simulink model "Furuta_Control_2015a"  (R2015a)
settings: Solver=ode3  SolverMode=SingleTasking  StartTime=0.0  StopTime=10  FixedStep=0.0001  RelTol=1e-3
PostLoadFcn:
  | , if any(exist('dsrtsu_mdlpostloadfcn', 'file') == [2, 3, 6]), try dsrtsu_mdlpostloadfcn('Execute', bdroot); catch fprintf('Error in PostLoadFcn (dsrtsu_mdlpostloadfcn) for model "%s":\n %s\n', bdroot, lasterr); end, end,
values from neighbouring files (symbols this model uses):
  alpha = J + (M+m1/3+m2)*L1^2    (= 0.002160093571)    [Furuta_Constants.m]
  beta = (M + m2/3)*L2^2    (= 0.00192796261667)    [Furuta_Constants.m]
  gamma = (M + m2/2)*L2*L1    (= 0.0009263333625)    [Furuta_Constants.m]
  initial_state = pi    (= 3.14159265359)    [Furuta_Constants.m]
  K = place(Ap,Bp,[-7 -5 -3+3j -3-3j])    [Furuta_Constants.m]
  kb = 6e-4    (= 0.0006)    [Furuta_Constants.m]
  ke = 0.182    [Furuta_Constants.m]
  kSU = 0.44    [Furuta_Constants.m]
  Re = 3.6    [Furuta_Constants.m]
  sigma = (M + m2/2)*g*L2    (= 0.0951054975)    [Furuta_Constants.m]
libraries: simulink_extras x1
settings Model: DSRTSU_INTERNAL_RTI_VER=450  DSRTSU_INTERNAL_RTI_TYPE=rti1006  DSRTSU_INTERNAL_RTIFPGA=40  CovMetricSettings=dwe  CovHtmlReporting=off  covSaveCumulativeToWorkspaceVar=off  CovSaveSingleToWorkspaceVar=off  CovExternalEMLEnable=on  Creator=Marcelo  LastModifiedBy=NSEE
settings SolverCC: ZeroCrossControl=DisableAll
settings DataIOCC: LimitDataPoints=off  SaveFormat=Dataset
settings OptimizationCC: BlockReduction=off  OptimizeBlockIOStorage=off  BufferReuse=off  GlobalBufferReuse=off  ExpressionFolding=off  LocalBlockOutputs=off
settings DebuggingCC: ParameterOverflowMsg=warning  SFUnexpectedBacktrackingDiag=error  SFNoUnconditionalDefaultTransitionDiag=error
settings HardwareCC: ProdBitPerPointer=64  ProdLargestAtomicFloat=Float  ProdIntDivRoundTo=Zero  ProdEndianess=LittleEndian  ProdHWDeviceType=Generic->Custom  TargetIntDivRoundTo=Zero  TargetEndianess=LittleEndian  TargetHWDeviceType=Generic->Custom
settings ModelReferenceCC: ModelReferenceMinAlgLoopOccurrences=on  PropagateSignalLabelsOutOfModel=on
settings RTWCC: SystemTargetFile=rti1006.tlc  MakeCommand=make_rti  TemplateMakefile=rti1006.tmf  Description=dSPACE DS1006 Hardware Platform
settings STFCustomTargetCC: GenerateSampleERTMain=off  ParMdlRefBuildCompliant=on  GeneratePreprocessorConditionals=Disable all  ERTCustomFileBanners=off  SupportNonInlinedSFcns=on  SupportVariableSizeSignals=off  MATLABClassNameForMDSCustomization=Simulink.SoftwareTarget.GRTCustomization  GRTInterface=on  SystemTargetFile=rti1006.tlc
settings GRTTargetCC: CompOptLevelCompliant=off  ConcurrentExecutionCompliant=off  CombineOutputUpdateFcns=off  MatFileLogging=off  CPPClassGenCompliant=off  GRTInterface=on  ExtModeMexFile=noextcomm

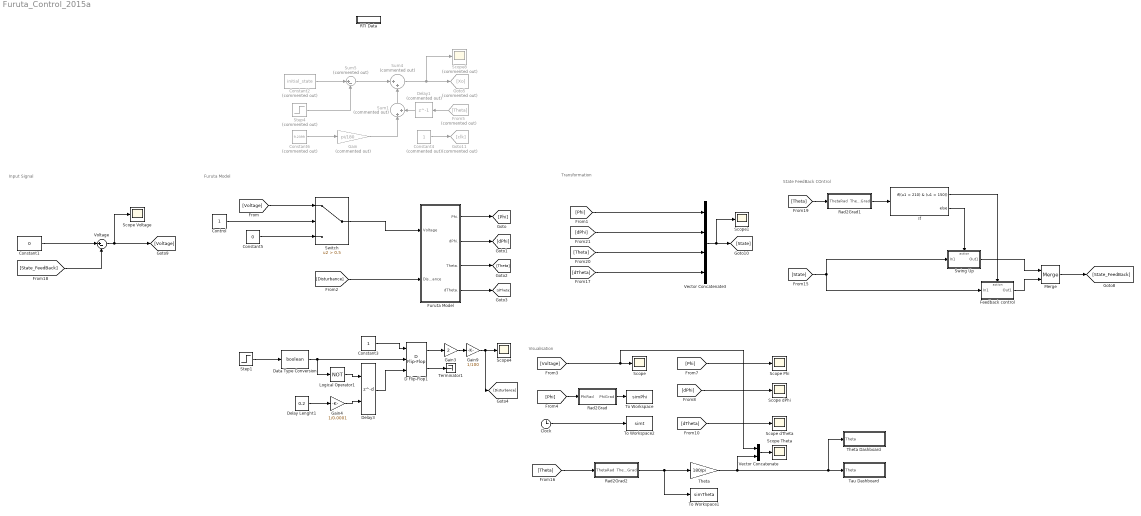
== system Furuta_Control_2015a ==
  note: Transformation
  note: State FeedBack COntrol
  note: Input Signal
  note: Furuta Model
  note: Visualisation
  Clock : Clock
  Constant1 : Constant  Value=0
  Constant2 : Constant  Commented=on  Value=initial_state
  Constant3 : Constant  OutDataTypeStr=boolean
  Constant4 : Constant  Commented=on
  Constant5 : Constant  Value=0
  Constant6 : Constant  Commented=on  Value=9.2399
  Control : Constant
  D Flip-Flop1 : simulink_extras/Flip Flops/D Flip-Flop
  Data Type Conversion : DataTypeConversion  OutDataTypeStr=boolean
  Delay Lenght1 : Constant  Value=0.2  OutDataTypeStr=double
  Delay1 : Delay  Commented=on  DelayLength=1
  Delay3 : Delay  DelayLengthSource=Input port  DelayLengthUpperLimit=100000  InitialCondition=1
      settings: InputPortMap=u0,p1
  Feedback control : Subsystem  TreatAsAtomicUnit=on
  From5 : From  Commented=on  GotoTag=Theta
  "Furuta Model " : Subsystem
  Gain : Gain  Commented=on  Gain=pi/180
  Gain3 : Gain  Gain=2  ParamDataTypeStr=double
  Gain4 : Gain  Gain=1/0.0001
  Gain9 : Gain  Gain=1/100
  Goto11 : Goto  Commented=on  GotoTag=clk
  Goto5 : Goto  Commented=on  GotoTag=Xo
  If : If  IfExpression=(u1 < 210) & (u1 > 150)
  Logical Operator1 : Logic  Operator=NOT  AllPortsSameDT=off  OutDataTypeStr=boolean
  Merge : Merge
  RTI Data : Subsystem  Tag=struct('RTIDataServer',struct('RTIDataServerVs','2','RTIModelDescription','struct(''main'',''Furuta_Control_2015a'',''sub'','''',''isMp'',0)'))  LoadFcn="if exist('rtidc'), try,  rtidc('DataHostBlockClbLoad', gcbh); catch, disp(['Warning: ''LoadFcn'' for RTI Data block failed: ' lasterr]); end, end,"  mask(RTI_DATA_HOST){}
      mask help:
      | RTI Data Block.
      | This block is used by RTI to store internal model-dependent data.
      | Please keep this block on the root level of the model. Deleting this block will result in data loss.
      |
      | NEVER DELETE OR COPY THIS BLOCK!
      settings: CopyFcn="if exist('rtidc'), try,  rtidc('DataHostBlockClbCopy', gcbh); catch, disp(['Warning: ''CopyFcn'' for RTI Data block failed: ' lasterr]); end, end,"  DeleteFcn="if exist('rtidc'), try,  rtidc('DataHostBlockClbDelete', gcbh); catch, disp(['Warning: ''DeleteFcn'' for RTI Data block failed: ' lasterr]); end, end,"  ModelCloseFcn="if exist('rtidc'), try,  rtidc('DataHostBlockClbModelClose', gcbh); catch, disp(['Warning: ''ModelCloseFcn'' for RTI Data block failed: ' lasterr]); end, end,"  PreSaveFcn="if exist('rtidc'), try,  rtidc('DataHostBlockClbPreSave', gcbh); catch, disp(['Warning: ''PreSaveFcn'' for RTI Data block failed: ' lasterr]); end, end,"  PostSaveFcn="if exist('rtidc'), try,  rtidc('DataHostBlockClbPostSave', gcbh); catch, disp(['Warning: ''PostSaveFcn'' for RTI Data block failed: ' lasterr]); end, end,"  NameChangeFcn="if exist('rtidc'), try,  rtidc('DataHostBlockClbNameChange', gcbh); catch, disp(['Warning: ''NameChangeFcn'' for RTI Data block failed: ' lasterr]); end, end,"
      mask Help:
      | RTI Data Block.
      | This block is used by RTI to store internal model-dependent data.
      | Please keep this block on the root level of the model. Deleting this block will result in data loss.
      | 
      | NEVER DELETE OR COPY THIS BLOCK!
      mask Display:
      | text(0.5, 0.5, 'RTI Data', 'HorizontalAlignment', 'center');
      | plot([1 0]);
  Rad2Grad : Subsystem
  Rad2Grad1 : Subsystem
  Rad2Grad2 : Subsystem
  Scope : Scope
      settings: YMin=-6.87803  YMax=6.87804
  Scope Phi : Scope
      settings: YMin=-2.67842  YMax=1.39934  SaveName=ScopeData4
  Scope Theta : Scope
      settings: TimeRange=10  YMin=-25  YMax=375  SaveName=ScopeData6
  Scope Voltage : Scope
      settings: YMin=-12.5  YMax=12.5
  Scope dPhi : Scope
      settings: YMin=-12.39064  YMax=9.91965  SaveName=ScopeData5
  Scope dTheta : Scope
      settings: YMin=-20.04064  YMax=17.40154  SaveName=ScopeData7
  Scope1 : Scope
      settings: YMin=-17.5  YMax=15  SaveName=ScopeData9
  Scope4 : Scope
      settings: YMin=0  YMax=0.0325  SaveName=ScopeData10
  Scope8 : Scope  Commented=on
      settings: SaveName=ScopeData8
  Step1 : Step  Time=7  SampleTime=0
  Step4 : Step  Commented=on  Time=0.5  After=initial_state  SampleTime=0
  Sum1 : Sum  Commented=on  Inputs=|++
  Sum4 : Sum  Commented=on  Inputs=|++
  Sum5 : Sum  Commented=on  Inputs=|+-
  Swing Up : Subsystem  TreatAsAtomicUnit=on
  Switch : Switch  Criteria=u2 > Threshold  Threshold=0.5
  Tau Dashboard : Subsystem
  Terminator1 : Terminator
  Theta : Gain  Gain=180/pi
  Theta Dashboard : Subsystem
  To Workspace : ToWorkspace  VariableName=simPhi  SampleTime=-1
      settings: Save2DSignal=2-D array (concatenate along first dimension)
  To Workspace1 : ToWorkspace  VariableName=simTheta  SampleTime=-1
      settings: Save2DSignal=2-D array (concatenate along first dimension)
  To Workspace2 : ToWorkspace  VariableName=simt  SampleTime=-1
      settings: Save2DSignal=2-D array (concatenate along first dimension)
  Vector Concatenate : Concatenate
  Vector Concatenate3 : Concatenate  NumInputs=4
  Voltage : Sum  Inputs=|+-
  wires:
  "Furuta Model "/1(Phi.) -> [Phi]
  "Furuta Model "/2(dPhi.) -> [dPhi]
  "Furuta Model "/3(Theta.) -> [Theta]
  [Voltage] -> Vector Concatenate/1, Scope/1
  [Phi] -> Scope Phi/1
  [dPhi] -> Scope dPhi/1
  [dTheta] -> Scope dTheta/1
  Constant1/1 -> Voltage/1
  [State_FeedBack] -> Voltage/2
  Voltage/1 -> Scope Voltage/1, [Voltage]
  [dPhi] -> Vector Concatenate3/2
  Vector Concatenate3/1 -> [State], Scope1/1
  [Theta] -> Vector Concatenate3/3
  [Phi] -> Rad2Grad/1(PhiRad)
  [Theta] -> Rad2Grad2/1(ThetaRad)
  Rad2Grad2/1(ThetaGrad) -> To Workspace1/1, Theta/1
  Clock/1 -> To Workspace2/1
  Rad2Grad/1(PhiGrad) -> To Workspace/1
  If/2 -> Swing Up/Action
  [State] -> Swing Up/1(In1), Feedback control/1(In1)
  Swing Up/1(Out1) -> Merge/1
  If/1 -> Feedback control/Action
  Theta/1 -> Vector Concatenate/2, Theta Dashboard/1(Theta), Tau Dashboard/1("Theta ")
  Rad2Grad1/1(ThetaGrad) -> If/1
  [Theta] -> Rad2Grad1/1(ThetaRad)
  "Furuta Model "/4(dTheta.) -> [dTheta]
  [dTheta] -> Vector Concatenate3/4
  Step4/1 -> Sum5/2
  Sum4/1 -> Scope8/1, Goto5/1
  Sum5/1 -> Sum4/1
  Constant2/1 -> Sum5/1
  Constant6/1 -> Gain/1
  [Voltage] -> Switch/1
  Control/1 -> Switch/2
  Constant5/1 -> Switch/3
  Constant4/1 -> Goto11/1
  From5/1 -> Delay1/1
  Gain/1 -> Sum1/1
  Sum1/1 -> Sum4/2
  Delay1/1 -> Sum1/2
  [Phi] -> Vector Concatenate3/1
  Vector Concatenate/1 -> Scope Theta/1
  Feedback control/1(Out1) -> Merge/2
  Merge/1 -> [State_FeedBack]
  Switch/1 -> "Furuta Model "/1("Voltage ")
  [Disturbance] -> "Furuta Model "/2(Disturbance)
  Constant3/1 -> D Flip-Flop1/1
  Delay3/1 -> D Flip-Flop1/3
  Logical Operator1/1 -> Delay3/1
  Step1/1 -> Data Type Conversion/1
  D Flip-Flop1/1 -> Gain3/1
  Gain3/1 -> Gain9/1
  D Flip-Flop1/2 -> Terminator1/1
  Delay Lenght1/1 -> Gain4/1
  Gain4/1 -> Delay3/2
  Data Type Conversion/1 -> Logical Operator1/1, D Flip-Flop1/2
  Gain9/1 -> [Disturbance], Scope4/1

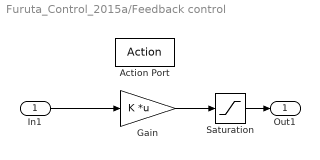
== system Furuta_Control_2015a/Feedback control ==
  In1 : Inport
  Action Port : ActionPort  ActionType=then
  Gain : Gain  Gain=K  Multiplication=Matrix(K*u)  ParamDataTypeStr=double  OutDataTypeStr=double
  Saturation : Saturate  UpperLimit=12  LowerLimit=-12
  Out1 : Outport
  wires:
  In1/1 -> Gain/1
  Gain/1 -> Saturation/1
  Saturation/1 -> Out1/1

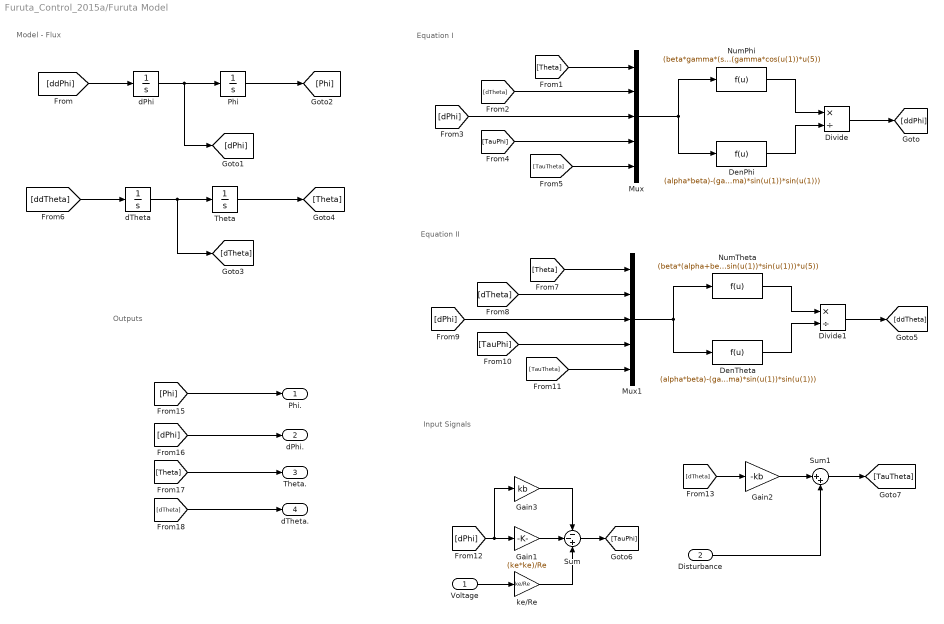
== system Furuta_Control_2015a/Furuta Model  ==
  note: Outputs
  note: Input Signals
  note: Equation II
  note: Equation I
  note: Model - Flux
  "Voltage " : Inport
  Disturbance : Inport  Port=2
  DenPhi : Fcn  Expr=(alpha*beta)-(gamma*gamma)+((beta*beta+gamma*gamma)*sin(u(1))*sin(u(1)))
  DenTheta : Fcn  Expr=(alpha*beta)-(gamma*gamma)+((beta*beta+gamma*gamma)*sin(u(1))*sin(u(1)))
  Divide : Product  Inputs=*/
  Divide1 : Product  Inputs=*/
  Gain1 : Gain  Gain=(ke*ke)/Re
  Gain2 : Gain  Gain=-kb
  Gain3 : Gain  Gain=kb
  Mux : Mux  Inputs=5
  Mux1 : Mux  Inputs=5
  NumPhi : Fcn  Expr=(beta*gamma*(sin(u(1))*sin(u(1))-1)*sin(u(1))*u(3)*u(3))-(2*beta*beta*cos(u(1))*sin(u(1))*u(3)*u(2))+(beta*gamma*sin(u(1))*u(2)*u(2))-(gamma*sigma*cos(u(1))*sin(u(1)))+(beta*u(4))-(gamma*cos(u(1))*u(5))
  NumTheta : Fcn  Expr=(beta*(alpha+beta*sin(u(1))*sin(u(1)))*cos(u(1))*sin(u(1))*u(3)*u(3))+(2*beta*gamma*(1-sin(u(1))*sin(u(1)))*sin(u(1))*u(3)*u(2))-(gamma*gamma*cos(u(1))*sin(u(1))*u(2)*u(2))+(sigma*(alpha+beta*sin(u(1))*sin(u(1)))*sin(u(1)))-(gamma*cos(u(1))*u(4))+((alpha+beta*sin(u(1))*sin(u(1)))*u(5))
  Phi : Integrator
  Sum : Sum  Inputs=--+
  Sum1 : Sum  Inputs=|++
  Theta : Integrator  InitialCondition=initial_state
  dPhi : Integrator
  dTheta : Integrator
  "ke/Re " : Gain  Gain=ke/Re
  Phi. : Outport
  dPhi. : Outport  Port=2
  Theta. : Outport  Port=3
  dTheta. : Outport  Port=4
  wires:
  Divide/1 -> [ddPhi]
  "ke/Re "/1 -> Sum/3
  Sum/1 -> [TauPhi]
  Gain1/1 -> Sum/2
  "Voltage "/1 -> "ke/Re "/1
  [dTheta] -> Gain2/1
  Gain3/1 -> Sum/1
  dTheta/1 -> [dTheta], Theta/1
  [Theta] -> Mux1/1
  Mux1/1 -> DenTheta/1, NumTheta/1
  [dTheta] -> Mux1/2
  [dPhi] -> Mux1/3
  [TauTheta] -> Mux1/5
  [TauPhi] -> Mux1/4
  [Theta] -> Mux/1
  [TauTheta] -> Mux/5
  [TauPhi] -> Mux/4
  Phi/1 -> [Phi]
  [dPhi] -> Mux/3
  DenPhi/1 -> Divide/2
  [ddPhi] -> dPhi/1
  [ddTheta] -> dTheta/1
  dPhi/1 -> [dPhi], Phi/1
  NumTheta/1 -> Divide1/1
  NumPhi/1 -> Divide/1
  DenTheta/1 -> Divide1/2
  Mux/1 -> DenPhi/1, NumPhi/1
  [dPhi] -> Gain3/1, Gain1/1
  [dTheta] -> Mux/2
  Divide1/1 -> [ddTheta]
  [Phi] -> Phi./1
  [dPhi] -> dPhi./1
  [Theta] -> Theta./1
  [dTheta] -> dTheta./1
  Theta/1 -> [Theta]
  Disturbance/1 -> Sum1/2
  Gain2/1 -> Sum1/1
  Sum1/1 -> [TauTheta]

== system Furuta_Control_2015a/RTI Data ==
  RTI Data Store : Subsystem  Tag="struct('private',struct('version',struct('dsVer',uint32(2),'dsVerCreation',uint32(2),'RTI',struct('ver','7.3','type','RTI1006')),'access',struct('type','Model','isPerm',1,'created',['02-Oct-2018 16:40:55'],'modified',['06-Nov-2018 22:49:19'],'location','')),'public',struct('main',struct('data',[]),'sub',struct('name',{{'Furuta_Control_2015a'}},'data',{{struct('TH',struct('thTaskInfo',struct('taskType',{'TIMER','HWINT','TMRINT','SWINT','GLINT'},'tasksNumOf',{1,0,0,0,0},'srcIds',{{'TIMERA'},{},{},{},{}},'taskNames',{{['Timer Task 1']},{},{},{},{}})),'th_tc',struct('dataType','TASK','taskGroupId','','taskGroupList',{{}},'taskSchedulingPolicy','FCFS','taskType','TIMER','blkh',-1,'srcId','TIMERA','srcSgnName',['Timer A interrupt'],'srcCpuName','','taskName',['Timer Task 1  [0.0001] s'],'taskNameDisplayExt','','smplTime',0.0001,'smplTimeOffs',0,'hasFixedPriority',0,'priority',1,'hasFixedOvc',0,'ovcType',1,'ovcMax',1),'tc_th',struct('dataType','TASK','taskGroupId','','taskGroupList',{{}},'taskSchedulingPolicy','FCFS','taskType','TIMER','blkh',-1,'srcId','TIMERA','srcSgnName',['Timer A interrupt'],'srcCpuName','','taskName',['Timer Task 1  [0.0001] s'],'taskNameDisplayExt','','smplTime',0.0001,'smplTimeOffs',0,'hasFixedPriority',0,'priority',1,'hasFixedOvc',0,'ovcType',1,'ovcMax',1))}})))"  mask(RTI_DATA_STORE){}
      mask help:
      | RTI Data Store Block. This block is used by RTI to store internal model dependent data. Deleting this block will result in data loss.
      |
      | NEVER DELETE, COPY, OR MODIFY THIS BLOCK!
      mask Help:
      | RTI Data Store Block. This block is used by RTI to store internal model dependent data. Deleting this block will result in data loss.
      | 
      | NEVER DELETE, COPY, OR MODIFY THIS BLOCK!
      mask Display: text(0.5, 0.5, ' ', 'HorizontalAlignment', 'center');

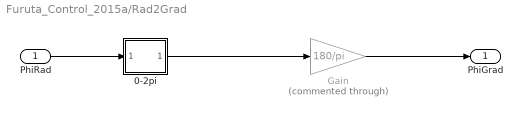
== system Furuta_Control_2015a/Rad2Grad ==
  PhiRad : Inport
  0-2pi : Subsystem
  Gain : Gain  Commented=through  Gain=180/pi
  PhiGrad : Outport
  wires:
  0-2pi/1(Out1) -> Gain/1
  Gain/1 -> PhiGrad/1
  PhiRad/1 -> 0-2pi/1(In1)

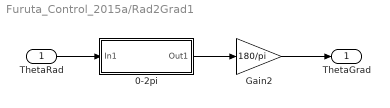
== system Furuta_Control_2015a/Rad2Grad1 ==
  ThetaRad : Inport
  0-2pi : Subsystem
  Gain2 : Gain  Gain=180/pi
  ThetaGrad : Outport
  wires:
  ThetaRad/1 -> 0-2pi/1(In1)
  0-2pi/1(Out1) -> Gain2/1
  Gain2/1 -> ThetaGrad/1

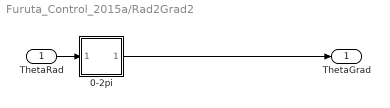
== system Furuta_Control_2015a/Rad2Grad2 ==
  ThetaRad : Inport
  0-2pi : Subsystem
  ThetaGrad : Outport
  wires:
  ThetaRad/1 -> 0-2pi/1(In1)
  0-2pi/1(Out1) -> ThetaGrad/1

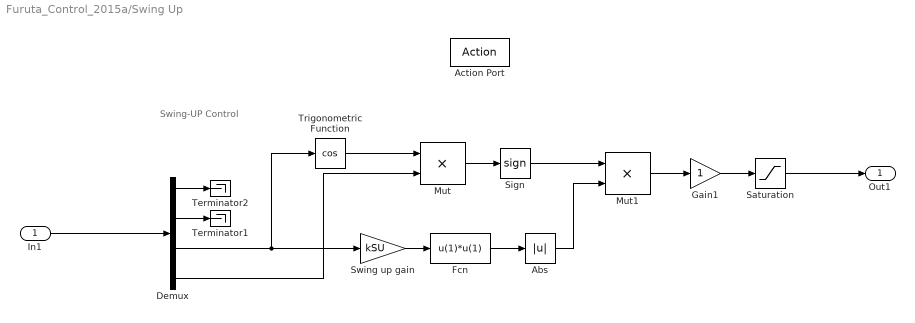
== system Furuta_Control_2015a/Swing Up ==
  note: Swing-UP Control
  In1 : Inport
  Action Port : ActionPort  ActionType=else
  Abs : Abs
  Demux : Demux
  Fcn : Fcn  Expr=u(1)*u(1)
  Gain1 : Gain
  Mut : Product  Inputs=**
  Mut1 : Product  Inputs=**
  Saturation : Saturate  UpperLimit=12  LowerLimit=-12
  Sign : Signum
  Swing up gain : Gain  Gain=kSU
  Terminator1 : Terminator
  Terminator2 : Terminator
  Trigonometric Function : Trigonometry  Operator=cos
  Out1 : Outport  InitialOutput=0
  wires:
  Saturation/1 -> Out1/1
  Demux/2 -> Terminator1/1
  Demux/1 -> Terminator2/1
  Gain1/1 -> Saturation/1
  Mut1/1 -> Gain1/1
  Demux/3 -> Trigonometric Function/1, Swing up gain/1
  Fcn/1 -> Abs/1
  Trigonometric Function/1 -> Mut/1
  Demux/4 -> Mut/2
  Abs/1 -> Mut1/2
  Sign/1 -> Mut1/1
  Mut/1 -> Sign/1
  Swing up gain/1 -> Fcn/1
  In1/1 -> Demux/1

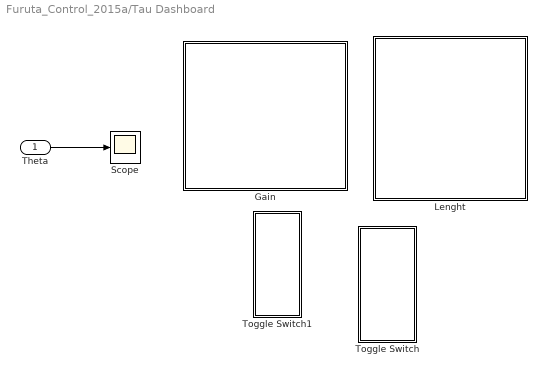
== system Furuta_Control_2015a/Tau Dashboard ==
  "Theta " : Inport
  Gain : Subsystem  DialogController=hmiCreateDDGDialog  IsWebBlock=on  mask(MathWorksWebBlock){webBlockId=4df3a667-03b8-4ac4-b39a-9a126b51fd8c, webBlockType=continuousknob, ShowInLibBrowser=on, ShowInitialText=on, HMISrcModelName=Furuta_Control_2015a}
      mask prompts: webBlockId "WebBlock Id"; webBlockType "WebBlock Type"; HMISrcModelName "Source Model"
      mask help: SimulinkHMI:dialogs:ContinuousKnobDialogDesc
      mask Help: helpview([docroot '/mapfiles/simulink.map'], 'hmi_knob')
      mask Display:
      | if strcmp(get_param(bdroot(gcb),'BlockDiagramType'), 'library')
      |     image([(matlabroot) '/toolbox/simulink/hmi/icons/ContinuousKnob.png']);
      | end
  Lenght : Subsystem  DialogController=hmiCreateDDGDialog  IsWebBlock=on  mask(MathWorksWebBlock){webBlockId=2ffdbfce-ad2c-4f82-8aaa-bb0c61bbc096, webBlockType=continuousknob, ShowInLibBrowser=on, ShowInitialText=on, HMISrcModelName=Furuta_Control_2015a}
      mask prompts: webBlockId "WebBlock Id"; webBlockType "WebBlock Type"; HMISrcModelName "Source Model"
      mask help: SimulinkHMI:dialogs:ContinuousKnobDialogDesc
      mask Help: helpview([docroot '/mapfiles/simulink.map'], 'hmi_knob')
      mask Display:
      | if strcmp(get_param(bdroot(gcb),'BlockDiagramType'), 'library')
      |     image([(matlabroot) '/toolbox/simulink/hmi/icons/ContinuousKnob.png']);
      | end
  Scope : Scope
      settings: TimeRange=10  YMin=0  YMax=375  SaveName=ScopeData2
  Toggle Switch : Subsystem  DialogController=hmiCreateDDGDialog  IsWebBlock=on  mask(MathWorksWebBlock){webBlockId=9ef78f83-ce25-4a6d-8579-1dd4683104fe, webBlockType=toggleswitch, ShowInLibBrowser=on, ShowInitialText=on, HMISrcModelName=Furuta_Control_2015a}
      mask prompts: webBlockId "WebBlock Id"; webBlockType "WebBlock Type"; HMISrcModelName "Source Model"
      mask help: SimulinkHMI:dialogs:SwitchDialogDesc
      mask Help: helpview([docroot '/mapfiles/simulink.map'], 'hmi_toggle_switch')
      mask Display:
      | if strcmp(get_param(bdroot(gcb),'BlockDiagramType'), 'library')
      |     image([(matlabroot) '/toolbox/simulink/hmi/icons/ToggleSwitch.png']);
      | end
  Toggle Switch1 : Subsystem  DialogController=hmiCreateDDGDialog  IsWebBlock=on  mask(MathWorksWebBlock){webBlockId=93f7e4e2-254a-49cd-95ec-091a15108054, webBlockType=toggleswitch, ShowInLibBrowser=on, ShowInitialText=on, HMISrcModelName=Furuta_Control_2015a}
      mask prompts: webBlockId "WebBlock Id"; webBlockType "WebBlock Type"; HMISrcModelName "Source Model"
      mask Help: helpview([docroot '/mapfiles/simulink.map'], 'hmi_toggle_switch')
      mask Display:
      | if strcmp(get_param(bdroot(gcb),'BlockDiagramType'), 'library')
      |     image([(matlabroot) '/toolbox/simulink/hmi/icons/ToggleSwitch.png']);
      | end
  wires:
  "Theta "/1 -> Scope/1

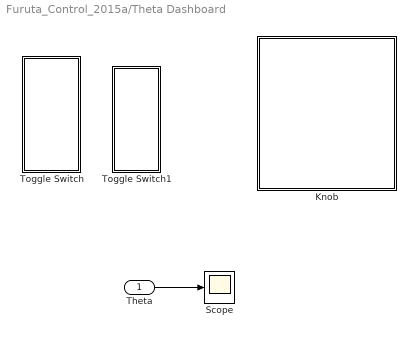
== system Furuta_Control_2015a/Theta Dashboard ==
  Theta : Inport
  Knob : Subsystem  DialogController=hmiCreateDDGDialog  IsWebBlock=on  mask(MathWorksWebBlock){webBlockId=aac29083-8fd0-4520-b4bd-68fb2bedaac5, webBlockType=continuousknob, ShowInLibBrowser=on, ShowInitialText=on, HMISrcModelName=Furuta_Control_2015a}
      mask prompts: webBlockId "WebBlock Id"; webBlockType "WebBlock Type"; HMISrcModelName "Source Model"
      mask help: SimulinkHMI:dialogs:ContinuousKnobDialogDesc
      mask Help: helpview([docroot '/mapfiles/simulink.map'], 'hmi_knob')
      mask Display:
      | if strcmp(get_param(bdroot(gcb),'BlockDiagramType'), 'library')
      |     image([(matlabroot) '/toolbox/simulink/hmi/icons/ContinuousKnob.png']);
      | end
  Scope : Scope
      settings: YMin=-44.99482  YMax=404.9865
  Toggle Switch : Subsystem  DialogController=hmiCreateDDGDialog  IsWebBlock=on  mask(MathWorksWebBlock){webBlockId=1ab1796d-89f8-4362-a8ce-2d672f8a6157, webBlockType=toggleswitch, ShowInLibBrowser=on, ShowInitialText=on, HMISrcModelName=Furuta_Control_2015a}
      mask prompts: webBlockId "WebBlock Id"; webBlockType "WebBlock Type"; HMISrcModelName "Source Model"
      mask help: SimulinkHMI:dialogs:SwitchDialogDesc
      mask Help: helpview([docroot '/mapfiles/simulink.map'], 'hmi_toggle_switch')
      mask Display:
      | if strcmp(get_param(bdroot(gcb),'BlockDiagramType'), 'library')
      |     image([(matlabroot) '/toolbox/simulink/hmi/icons/ToggleSwitch.png']);
      | end
  Toggle Switch1 : Subsystem  DialogController=hmiCreateDDGDialog  IsWebBlock=on  mask(MathWorksWebBlock){webBlockId=3e63f1bc-ff51-4ae5-8a6d-5f4cc210e1c8, webBlockType=toggleswitch, ShowInLibBrowser=on, ShowInitialText=on, HMISrcModelName=Furuta_Control_2015a}
      mask prompts: webBlockId "WebBlock Id"; webBlockType "WebBlock Type"; HMISrcModelName "Source Model"
      mask Help: helpview([docroot '/mapfiles/simulink.map'], 'hmi_toggle_switch')
      mask Display:
      | if strcmp(get_param(bdroot(gcb),'BlockDiagramType'), 'library')
      |     image([(matlabroot) '/toolbox/simulink/hmi/icons/ToggleSwitch.png']);
      | end
  wires:
  Theta/1 -> Scope/1

== system Furuta_Control_2015a/RTI Data/RTI Data Store ==
  RTI Data Store : Subsystem  mask(RTI_DATA_STORE){}
      mask help:
      | RTI Data Store Block. This block is used by RTI to store internal model dependent data. Deleting this block will result in data loss.
      |
      | NEVER DELETE, COPY, OR MODIFY THIS BLOCK!
      mask Help:
      | RTI Data Store Block. This block is used by RTI to store internal model dependent data. Deleting this block will result in data loss.
      | 
      | NEVER DELETE, COPY, OR MODIFY THIS BLOCK!
      mask Display: text(0.5, 0.5, ' ', 'HorizontalAlignment', 'center');

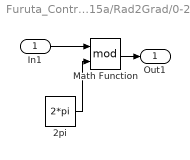
== system Furuta_Control_2015a/Rad2Grad/0-2pi ==
  In1 : Inport
  2pi : Constant  Value=2*pi
  Math Function : Math  Operator=mod  SaturateOnIntegerOverflow=on
  Out1 : Outport
  wires:
  2pi/1 -> Math Function/2
  Math Function/1 -> Out1/1
  In1/1 -> Math Function/1

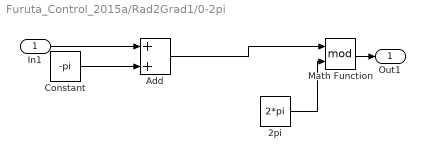
== system Furuta_Control_2015a/Rad2Grad1/0-2pi ==
  In1 : Inport
  2pi : Constant  Value=2*pi
  Add : Sum
  Constant : Constant  Value=-pi
  Math Function : Math  Operator=mod  SaturateOnIntegerOverflow=on
  Out1 : Outport
  wires:
  Math Function/1 -> Out1/1
  2pi/1 -> Math Function/2
  Constant/1 -> Add/2
  In1/1 -> Add/1
  Add/1 -> Math Function/1

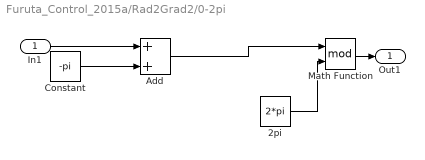
== system Furuta_Control_2015a/Rad2Grad2/0-2pi ==
  In1 : Inport
  2pi : Constant  Value=2*pi
  Add : Sum
  Constant : Constant  Value=-pi
  Math Function : Math  Operator=mod  SaturateOnIntegerOverflow=on
  Out1 : Outport
  wires:
  Math Function/1 -> Out1/1
  2pi/1 -> Math Function/2
  Constant/1 -> Add/2
  In1/1 -> Add/1
  Add/1 -> Math Function/1

== system Furuta_Control_2015a/Tau Dashboard/Gain ==

== system Furuta_Control_2015a/Tau Dashboard/Lenght ==

== system Furuta_Control_2015a/Tau Dashboard/Toggle Switch ==

== system Furuta_Control_2015a/Tau Dashboard/Toggle Switch1 ==

== system Furuta_Control_2015a/Theta Dashboard/Knob ==

== system Furuta_Control_2015a/Theta Dashboard/Toggle Switch ==

== system Furuta_Control_2015a/Theta Dashboard/Toggle Switch1 ==

== system Furuta_Control_2015a/RTI Data/RTI Data Store/RTI Data Store ==
  RTI Data Store : Subsystem  mask(RTI_DATA_STORE){}
      mask help:
      | RTI Data Store Block. This block is used by RTI to store internal model dependent data. Deleting this block will result in data loss.
      |
      | NEVER DELETE, COPY, OR MODIFY THIS BLOCK!
      mask Help:
      | RTI Data Store Block. This block is used by RTI to store internal model dependent data. Deleting this block will result in data loss.
      | 
      | NEVER DELETE, COPY, OR MODIFY THIS BLOCK!
      mask Display: text(0.5, 0.5, ' ', 'HorizontalAlignment', 'center');

== system Furuta_Control_2015a/RTI Data/RTI Data Store/RTI Data Store/RTI Data Store ==
  RTI Data Store : Subsystem  mask(RTI_DATA_STORE){}
      mask help:
      | RTI Data Store Block. This block is used by RTI to store internal model dependent data. Deleting this block will result in data loss.
      |
      | NEVER DELETE, COPY, OR MODIFY THIS BLOCK!
      mask Help:
      | RTI Data Store Block. This block is used by RTI to store internal model dependent data. Deleting this block will result in data loss.
      | 
      | NEVER DELETE, COPY, OR MODIFY THIS BLOCK!
      mask Display: text(0.5, 0.5, ' ', 'HorizontalAlignment', 'center');

== system Furuta_Control_2015a/RTI Data/RTI Data Store/RTI Data Store/RTI Data Store/RTI Data Store ==
